simulink model "satelliteSim"  (R2013b)
settings: Solver=ode45  StartTime=0.0  StopTime=10.0  RelTol=1e-3
values from neighbouring files (symbols this model uses):
  disturbance = 10000    [satellite.m]    (also in satelliteGUI.m = str2double(disturbance))
  I = 20    [satellite.m]    (also in satelliteGUI.m = str2double(I))
  J = 2    [satellite.m]    (also in satelliteGUI.m)
  Jhat = 1    [satellite.m]    (also in satelliteGUI.m)
  mud = 10    [satellite.m]    (also in satelliteGUI.m)
  mup = 10    [satellite.m]    (also in satelliteGUI.m)
  thetar = r    (= 1)    [satellite.m]    (also in satelliteGUI.m)
  thetardot = 0    [satellite.m]    (also in satelliteGUI.m)
  wn = 10    [satellite.m]    (also in satelliteGUI.m)
  zeta = 1    [satellite.m]    (also in satelliteGUI.m)
settings Model: Creator=Kristina  LastModifiedBy=Kristina

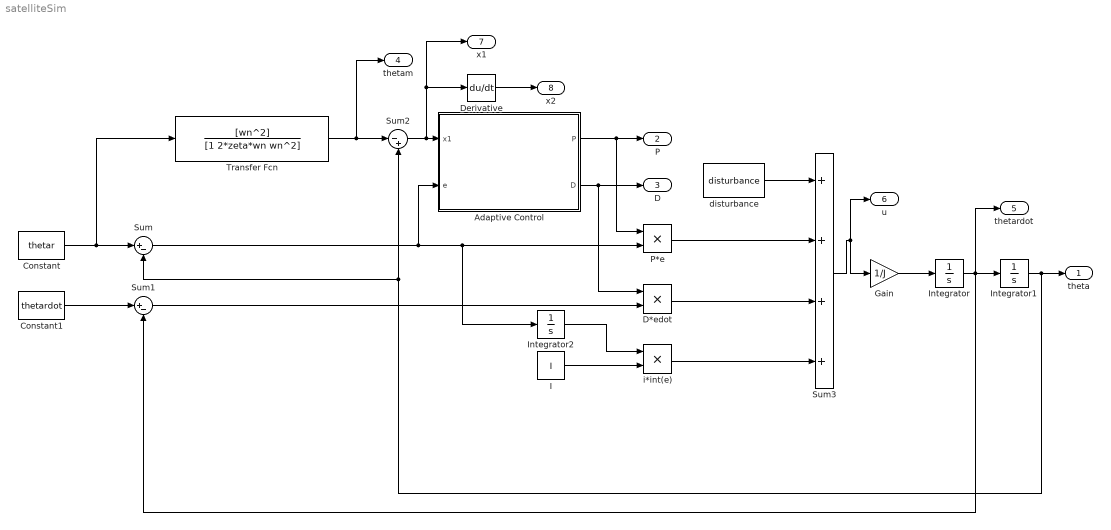
== system satelliteSim ==
  Adaptive Control : Subsystem
  Constant : Constant  Value=thetar
  Constant1 : Constant  Value=thetardot
  D*edot : Product
  Derivative : Derivative
  Gain : Gain  Gain=1/J
  I : Constant  Value=I
  Integrator : Integrator
  Integrator1 : Integrator
  Integrator2 : Integrator
  P*e : Product
  Sum : Sum  Inputs=|+-
  Sum1 : Sum  Inputs=|+-
  Sum2 : Sum  Inputs=|-+
  Sum3 : Sum  Inputs=++++
  Transfer Fcn : TransferFcn  Numerator=[wn^2]  Denominator=[1 2*zeta*wn wn^2]
  disturbance : Constant  Value=disturbance
  i*int(e) : Product
  theta : Outport
  P : Outport  Port=2
  D : Outport  Port=3
  thetam : Outport  Port=4
  thetardot : Outport  Port=5
  u : Outport  Port=6
  x1 : Outport  Port=7
  x2 : Outport  Port=8
  wires:
  Constant/1 -> Transfer Fcn/1, Sum/1
  Constant1/1 -> Sum1/1
  Sum/1 -> Adaptive Control/2(e), Integrator2/1, P*e/2
  Adaptive Control/1(P) -> P*e/1, P/1
  Adaptive Control/2(D) -> D*edot/1, D/1
  Sum1/1 -> D*edot/2
  D*edot/1 -> Sum3/3
  P*e/1 -> Sum3/2
  Sum3/1 -> Gain/1, u/1
  Gain/1 -> Integrator/1
  Integrator/1 -> thetardot/1, Integrator1/1, Sum1/2
  Integrator1/1 -> Sum/2, Sum2/2, theta/1
  Transfer Fcn/1 -> thetam/1, Sum2/1
  Sum2/1 -> Derivative/1, x1/1, Adaptive Control/1(x1)
  Derivative/1 -> x2/1
  disturbance/1 -> Sum3/1
  I/1 -> i*int(e)/2
  Integrator2/1 -> i*int(e)/1
  i*int(e)/1 -> Sum3/4

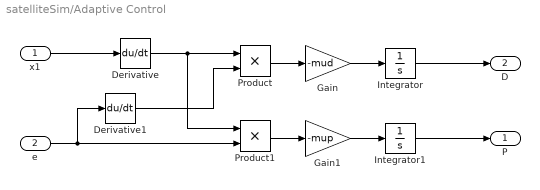
== system satelliteSim/Adaptive Control ==
  x1 : Inport
  e : Inport  Port=2
  Derivative : Derivative
  Derivative1 : Derivative
  Gain : Gain  Gain=-mud
  Gain1 : Gain  Gain=-mup
  Integrator : Integrator  InitialCondition=Jhat*2*zeta*wn
  Integrator1 : Integrator  InitialCondition=Jhat*wn^2
  Product : Product
  Product1 : Product
  P : Outport
  D : Outport  Port=2
  wires:
  Integrator1/1 -> P/1
  x1/1 -> Derivative/1
  e/1 -> Product1/2, Derivative1/1
  Product/1 -> Gain/1
  Integrator/1 -> D/1
  Derivative/1 -> Product1/1, Product/1
  Gain1/1 -> Integrator1/1
  Derivative1/1 -> Product/2
  Product1/1 -> Gain1/1
  Gain/1 -> Integrator/1
